simulink model "Hires"  (Simulink 10.0)
settings: Solver=ode45  StartTime=0.0  StopTime=320  RelTol=1e-3  EnableMultiTasking=on
settings Model: Creator=UX31  LastModifiedBy=unknown
settings DataIOCC: LimitDataPoints=on
settings DebuggingCC: UnderspecifiedInitializationDetection=Simplified  MergeDetectMultiDrivingBlocksExec=error  SolverPrmCheckMsg=warning
settings GRTTargetCC: GeneratePreprocessorConditionals=Disable all  CombineOutputUpdateFcns=on  GRTInterface=off
settings ConfigComp: CovExternalEMLEnable=off  CovSFcnEnable=off

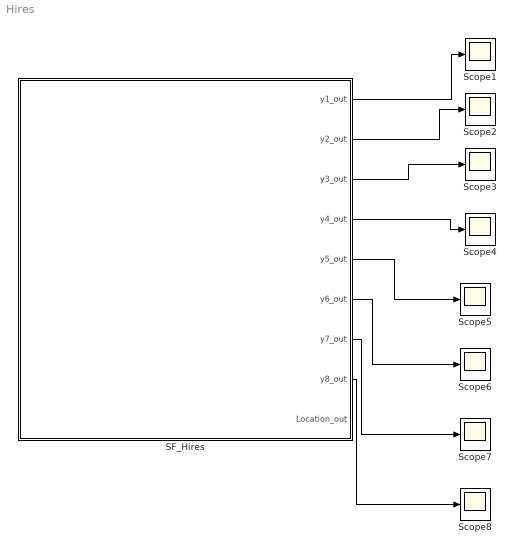
== system Hires ==
  SF_Hires : Stateflow chart  TreatAsAtomicUnit=on
  Scope{1..8} (8 alike) : Scope
  wires:
  SF_Hires/1(y1_out) -> Scope1/1
  SF_Hires/2(y2_out) -> Scope2/1
  SF_Hires/3(y3_out) -> Scope3/1
  SF_Hires/4(y4_out) -> Scope4/1
  SF_Hires/5(y5_out) -> Scope5/1
  SF_Hires/6(y6_out) -> Scope6/1
  SF_Hires/7(y7_out) -> Scope7/1
  SF_Hires/8(y8_out) -> Scope8/1

== stateflow chart SF_Hires ==
  settings: updateMethod=CONTINUOUS
  state always
    du:
    y1_dot=-1.71*y1+.43*y2+8.32*y3+0.0007;
    y2_dot=1.71*y1-8.75*y2;
    y3_dot=-10.03*y3+.43*y4+0.035*y5;
    y4_dot=8.32*y2+1.71*y3-1.12*y4;
    y5_dot=-1.745*y5+0.43*y6+0.43*y7;
    y6_dot=-280*y6*y8+0.69*y4+1.71*y5-0.43*y6+0.69*y7;
    y7_dot=280*y6*y8-1.81*y7;
    y8_dot=-280*y6*y8+1.81*y7;
    y1_out=y1;
    y2_out=y2;
    y3_out=y3;
    y4_out=y4;
    y5_out=y5;
    y6_out=y6;
    y7_out=y7;
    y8_out=y8;
    Location_out =1;
  (default) -> always : {y1=1;y2=0;y3=0;y4=0;y5=0;y6=0;y7=0;y8=0.0057}
  data: y1 local double; y1_out output double; y2 local double; y2_out output double; y3 local double; y3_out output double; y4 local double; y4_out output double; y5 local double; y5_out output double; y6 local double; y6_out output double; y7 local double; y7_out output double; y8 local double; y8_out output double; Location_out output double
  data y1 settings: updateMethod=SF_CONTINUOUS_TIME_DATA
  data y2 settings: updateMethod=SF_CONTINUOUS_TIME_DATA
  data y3 settings: updateMethod=SF_CONTINUOUS_TIME_DATA
  data y4 settings: updateMethod=SF_CONTINUOUS_TIME_DATA
  data y5 settings: updateMethod=SF_CONTINUOUS_TIME_DATA
  data y6 settings: updateMethod=SF_CONTINUOUS_TIME_DATA
  data y7 settings: updateMethod=SF_CONTINUOUS_TIME_DATA
  data y8 settings: updateMethod=SF_CONTINUOUS_TIME_DATA
